simulink model "gain_output_controller_sim"  (R2020b)
settings: Solver=FixedStepAuto  StartTime=0.0  StopTime=stop_time  RelTol=1e-3
InitFcn:
  | gain_output_controller_sim_init
StopFcn:
  | gain_output_controller_sim_stop
values from neighbouring files (symbols this model uses):
  fs = audio_fs * fft_up_sample_rate    (= 6144000)    [gain_output_controller_sim_init.m]
settings Model: Creator=t96f346  LastModifiedBy=conno
settings DataIOCC: ReturnWorkspaceOutputs=off

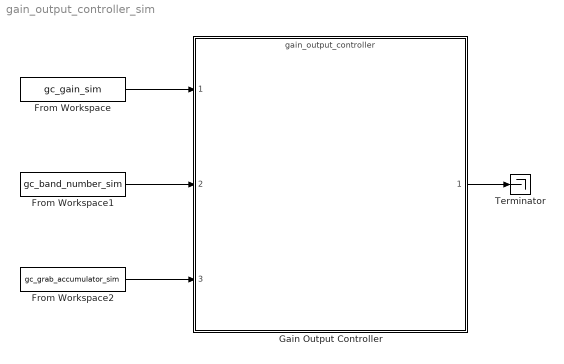
== system gain_output_controller_sim ==
  From Workspace : FromWorkspace  VariableName=gc_gain_sim  SampleTime=1/fs  Interpolate=off  OutputAfterFinalValue=Holding final value
  From Workspace1 : FromWorkspace  VariableName=gc_band_number_sim  SampleTime=-1  Interpolate=off  OutputAfterFinalValue=Holding final value
  From Workspace2 : FromWorkspace  VariableName=gc_grab_accumulator_sim  SampleTime=-1  Interpolate=off  OutputAfterFinalValue=Holding final value
  Gain Output Controller : ModelReference  ModelNameDialog=gain_output_controller.slx  SimulationMode=Normal  ModelReferenceVersion=2.35
  Terminator : Terminator
  wires:
  Gain Output Controller/1 -> Terminator/1
  From Workspace/1 -> Gain Output Controller/1
  From Workspace1/1 -> Gain Output Controller/2
  From Workspace2/1 -> Gain Output Controller/3
